simulink model "Hybrid_control_pid_final"  (R2021a)
settings: Solver=ode4  StartTime=0.0  StopTime=2+dt  FixedStep=dt  RelTol=1e-3
libraries: slpidlib x4
settings Model: Creator=Ashut  LastModifiedBy=Ashut

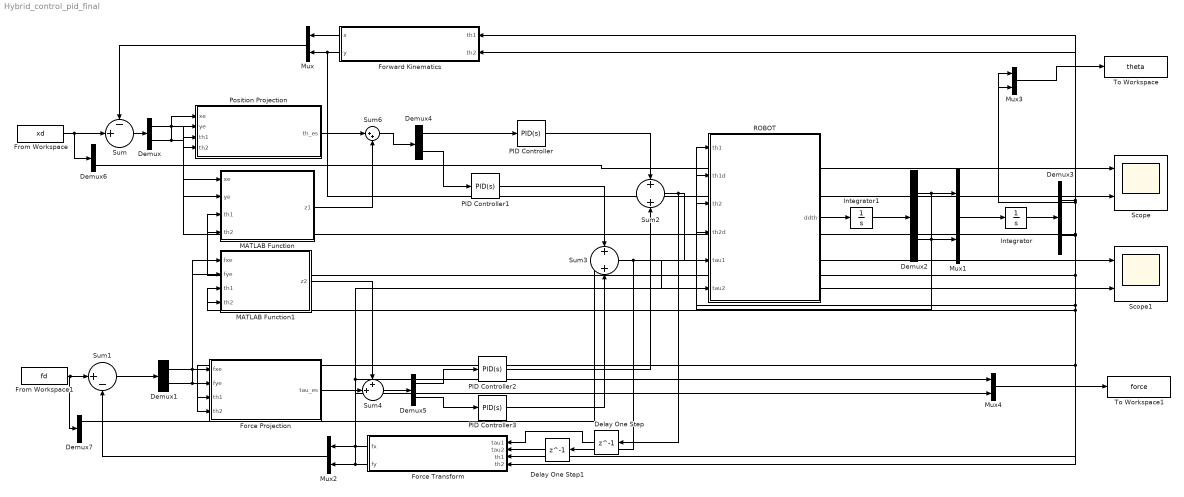
== system Hybrid_control_pid_final ==
  Delay One Step : Delay  DelayLength=1
  Delay One Step1 : Delay  DelayLength=1
  Demux{,1..7} (8 alike) : Demux  Outputs=2
  Force Projection : MATLAB Function  TreatAsAtomicUnit=on
  Force Transform : MATLAB Function  TreatAsAtomicUnit=on
  Forward Kinematics : MATLAB Function  TreatAsAtomicUnit=on
  From Workspace : FromWorkspace  VariableName=xd
  From Workspace1 : FromWorkspace  VariableName=fd
  Integrator : Integrator  InitialCondition=[-pi/3;0]
  Integrator1 : Integrator  InitialCondition=[0;0]
  MATLAB Function : MATLAB Function  TreatAsAtomicUnit=on
  MATLAB Function1 : MATLAB Function  TreatAsAtomicUnit=on
  Mux{,1..4} (5 alike) : Mux  Inputs=2
  PID Controller : slpidlib/PID Controller  Controller=PID  Form=Ideal  TimeDomain=Continuous-time  UseExternalTs=off  SampleTime=-1  IntegratorMethod=Forward Euler  FilterMethod=Forward Euler  ControllerParametersSource=internal  P=1  I=1  D=0  UseFilter=on  N=100  TunerSelectOption=Frequency Response Based  InitialConditionSource=internal  InitialConditionForIntegrator=0  InitialConditionForFilter=0  DifferentiatorICPrevScaledInput=0  ExternalReset=none  TrackingMode=off  Kt=1  LimitOutput=off  SatLimitsSource=internal  UpperSaturationLimit=inf  LowerSaturationLimit=-inf  LinearizeAsGain=on  AntiWindupMode=none  Kb=1  POutMin=[]  POutMax=[]  IOutMin=[]  IOutMax=[]  DOutMin=[]  DOutMax=[]  NOutMin=[]  NOutMax=[]  SumOutMin=[]  SumOutMax=[]  SaturationOutMin=[]  SaturationOutMax=[]  PParamMin=[]  PParamMax=[]  IParamMin=[]  IParamMax=[]  DParamMin=[]  DParamMax=[]  NParamMin=[]  NParamMax=[]  KbParamMin=[]  KbParamMax=[]  KtParamMin=[]  KtParamMax=[]  KbOutMin=[]  KbOutMax=[]  KtOutMin=[]  KtOutMax=[]  IntegratorOutMin=[]  IntegratorOutMax=[]  FilterOutMin=[]  FilterOutMax=[]  SumI1OutMin=[]  SumI1OutMax=[]  SumI2OutMin=[]  SumI2OutMax=[]  SumI3OutMin=[]  SumI3OutMax=[]  SumI4OutMin=[]  SumI4OutMax=[]  SumDOutMin=[]  SumDOutMax=[]  DifferentiatorOutMin=[]  DifferentiatorOutMax=[]  FilterDiffOutCoefMin=[]  FilterDiffOutCoefMax=[]  ReciprocalOutMin=[]  ReciprocalOutMax=[]  SumDenOutMin=[]  SumDenOutMax=[]  SumNumOutMin=[]  SumNumOutMax=[]  DivideOutMin=[]  DivideOutMax=[]  UdiffTsProdOutMin=[]  UdiffTsProdOutMax=[]  NTsProdOutMin=[]  NTsProdOutMax=[]  UintegralTsProdOutMin=[]  UintegralTsProdOutMax=[]  UngainTsProdOutMin=[]  UngainTsProdOutMax=[]  IntegratorContinuousStateAttributes=''  IntegratorStateMustResolveToSignalObject=off  IntegratorRTWStateStorageClass=Auto  FilterContinuousStateAttributes=''  FilterStateMustResolveToSignalObject=off  FilterRTWStateStorageClass=Auto  ParallelPVariant=Passthrough  IdealPVariant=InternalParameters  IVariant=InternalParameters  DVariant=InternalParameters  IntegratorVariant=Continuous  SatVariant=Disabled  AWVariant=Passthrough  PCopyVariant=Disabled  TRVariant=Disabled  FdbkBlocksVariant=Forward  IdealPFdbkVariant=Disabled  SatFdbkVariant=Disabled  DerivativeFilterVariant=ContFilter  NVariant=InternalParameters  NCopyVariant=Disabled  FilterICVariant=InternalICsFilter  IntegratorICVariant=InternalICs  ExternalResetVariant=Disabled  TRSumVariant=Passthrough  SumFdbkVariant=Disabled  SumVariant=Sum_PID  TsampFilterVariant=InternalTs  TsampNgainVariant=Passthrough  TsampIntegralVariant=Passthrough  ExternalSaturationOutDataTypeStr=Inherit: Same as second input
  PID Controller1 : slpidlib/PID Controller  Controller=PID  Form=Ideal  TimeDomain=Continuous-time  UseExternalTs=off  SampleTime=-1  IntegratorMethod=Forward Euler  FilterMethod=Forward Euler  ControllerParametersSource=internal  P=1  I=1  D=0  UseFilter=on  N=100  TunerSelectOption=Transfer Function Based (PID Tuner App)  InitialConditionSource=internal  InitialConditionForIntegrator=0  InitialConditionForFilter=0  DifferentiatorICPrevScaledInput=0  ExternalReset=none  TrackingMode=off  Kt=1  LimitOutput=off  SatLimitsSource=internal  UpperSaturationLimit=inf  LowerSaturationLimit=-inf  LinearizeAsGain=on  AntiWindupMode=none  Kb=1  POutMin=[]  POutMax=[]  IOutMin=[]  IOutMax=[]  DOutMin=[]  DOutMax=[]  NOutMin=[]  NOutMax=[]  SumOutMin=[]  SumOutMax=[]  SaturationOutMin=[]  SaturationOutMax=[]  PParamMin=[]  PParamMax=[]  IParamMin=[]  IParamMax=[]  DParamMin=[]  DParamMax=[]  NParamMin=[]  NParamMax=[]  KbParamMin=[]  KbParamMax=[]  KtParamMin=[]  KtParamMax=[]  KbOutMin=[]  KbOutMax=[]  KtOutMin=[]  KtOutMax=[]  IntegratorOutMin=[]  IntegratorOutMax=[]  FilterOutMin=[]  FilterOutMax=[]  SumI1OutMin=[]  SumI1OutMax=[]  SumI2OutMin=[]  SumI2OutMax=[]  SumI3OutMin=[]  SumI3OutMax=[]  SumI4OutMin=[]  SumI4OutMax=[]  SumDOutMin=[]  SumDOutMax=[]  DifferentiatorOutMin=[]  DifferentiatorOutMax=[]  FilterDiffOutCoefMin=[]  FilterDiffOutCoefMax=[]  ReciprocalOutMin=[]  ReciprocalOutMax=[]  SumDenOutMin=[]  SumDenOutMax=[]  SumNumOutMin=[]  SumNumOutMax=[]  DivideOutMin=[]  DivideOutMax=[]  UdiffTsProdOutMin=[]  UdiffTsProdOutMax=[]  NTsProdOutMin=[]  NTsProdOutMax=[]  UintegralTsProdOutMin=[]  UintegralTsProdOutMax=[]  UngainTsProdOutMin=[]  UngainTsProdOutMax=[]  IntegratorContinuousStateAttributes=''  IntegratorStateMustResolveToSignalObject=off  IntegratorRTWStateStorageClass=Auto  FilterContinuousStateAttributes=''  FilterStateMustResolveToSignalObject=off  FilterRTWStateStorageClass=Auto  ParallelPVariant=Passthrough  IdealPVariant=InternalParameters  IVariant=InternalParameters  DVariant=InternalParameters  IntegratorVariant=Continuous  SatVariant=Disabled  AWVariant=Passthrough  PCopyVariant=Disabled  TRVariant=Disabled  FdbkBlocksVariant=Forward  IdealPFdbkVariant=Disabled  SatFdbkVariant=Disabled  DerivativeFilterVariant=ContFilter  NVariant=InternalParameters  NCopyVariant=Disabled  FilterICVariant=InternalICsFilter  IntegratorICVariant=InternalICs  ExternalResetVariant=Disabled  TRSumVariant=Passthrough  SumFdbkVariant=Disabled  SumVariant=Sum_PID  TsampFilterVariant=InternalTs  TsampNgainVariant=Passthrough  TsampIntegralVariant=Passthrough  ExternalSaturationOutDataTypeStr=Inherit: Same as second input
  PID Controller2 : slpidlib/PID Controller  Controller=PID  Form=Ideal  TimeDomain=Continuous-time  UseExternalTs=off  SampleTime=-1  IntegratorMethod=Forward Euler  FilterMethod=Forward Euler  ControllerParametersSource=internal  P=1  I=1  D=0  UseFilter=on  N=100  TunerSelectOption=Transfer Function Based (PID Tuner App)  InitialConditionSource=internal  InitialConditionForIntegrator=0  InitialConditionForFilter=0  DifferentiatorICPrevScaledInput=0  ExternalReset=none  TrackingMode=off  Kt=1  LimitOutput=off  SatLimitsSource=internal  UpperSaturationLimit=inf  LowerSaturationLimit=-inf  LinearizeAsGain=on  AntiWindupMode=none  Kb=1  POutMin=[]  POutMax=[]  IOutMin=[]  IOutMax=[]  DOutMin=[]  DOutMax=[]  NOutMin=[]  NOutMax=[]  SumOutMin=[]  SumOutMax=[]  SaturationOutMin=[]  SaturationOutMax=[]  PParamMin=[]  PParamMax=[]  IParamMin=[]  IParamMax=[]  DParamMin=[]  DParamMax=[]  NParamMin=[]  NParamMax=[]  KbParamMin=[]  KbParamMax=[]  KtParamMin=[]  KtParamMax=[]  KbOutMin=[]  KbOutMax=[]  KtOutMin=[]  KtOutMax=[]  IntegratorOutMin=[]  IntegratorOutMax=[]  FilterOutMin=[]  FilterOutMax=[]  SumI1OutMin=[]  SumI1OutMax=[]  SumI2OutMin=[]  SumI2OutMax=[]  SumI3OutMin=[]  SumI3OutMax=[]  SumI4OutMin=[]  SumI4OutMax=[]  SumDOutMin=[]  SumDOutMax=[]  DifferentiatorOutMin=[]  DifferentiatorOutMax=[]  FilterDiffOutCoefMin=[]  FilterDiffOutCoefMax=[]  ReciprocalOutMin=[]  ReciprocalOutMax=[]  SumDenOutMin=[]  SumDenOutMax=[]  SumNumOutMin=[]  SumNumOutMax=[]  DivideOutMin=[]  DivideOutMax=[]  UdiffTsProdOutMin=[]  UdiffTsProdOutMax=[]  NTsProdOutMin=[]  NTsProdOutMax=[]  UintegralTsProdOutMin=[]  UintegralTsProdOutMax=[]  UngainTsProdOutMin=[]  UngainTsProdOutMax=[]  IntegratorContinuousStateAttributes=''  IntegratorStateMustResolveToSignalObject=off  IntegratorRTWStateStorageClass=Auto  FilterContinuousStateAttributes=''  FilterStateMustResolveToSignalObject=off  FilterRTWStateStorageClass=Auto  ParallelPVariant=Passthrough  IdealPVariant=InternalParameters  IVariant=InternalParameters  DVariant=InternalParameters  IntegratorVariant=Continuous  SatVariant=Disabled  AWVariant=Passthrough  PCopyVariant=Disabled  TRVariant=Disabled  FdbkBlocksVariant=Forward  IdealPFdbkVariant=Disabled  SatFdbkVariant=Disabled  DerivativeFilterVariant=ContFilter  NVariant=InternalParameters  NCopyVariant=Disabled  FilterICVariant=InternalICsFilter  IntegratorICVariant=InternalICs  ExternalResetVariant=Disabled  TRSumVariant=Passthrough  SumFdbkVariant=Disabled  SumVariant=Sum_PID  TsampFilterVariant=InternalTs  TsampNgainVariant=Passthrough  TsampIntegralVariant=Passthrough  ExternalSaturationOutDataTypeStr=Inherit: Same as second input
  PID Controller3 : slpidlib/PID Controller  Controller=PID  Form=Ideal  TimeDomain=Continuous-time  UseExternalTs=off  SampleTime=-1  IntegratorMethod=Forward Euler  FilterMethod=Forward Euler  ControllerParametersSource=internal  P=1  I=1  D=0  UseFilter=on  N=100  TunerSelectOption=Transfer Function Based (PID Tuner App)  InitialConditionSource=internal  InitialConditionForIntegrator=0  InitialConditionForFilter=0  DifferentiatorICPrevScaledInput=0  ExternalReset=none  TrackingMode=off  Kt=1  LimitOutput=off  SatLimitsSource=internal  UpperSaturationLimit=inf  LowerSaturationLimit=-inf  LinearizeAsGain=on  AntiWindupMode=none  Kb=1  POutMin=[]  POutMax=[]  IOutMin=[]  IOutMax=[]  DOutMin=[]  DOutMax=[]  NOutMin=[]  NOutMax=[]  SumOutMin=[]  SumOutMax=[]  SaturationOutMin=[]  SaturationOutMax=[]  PParamMin=[]  PParamMax=[]  IParamMin=[]  IParamMax=[]  DParamMin=[]  DParamMax=[]  NParamMin=[]  NParamMax=[]  KbParamMin=[]  KbParamMax=[]  KtParamMin=[]  KtParamMax=[]  KbOutMin=[]  KbOutMax=[]  KtOutMin=[]  KtOutMax=[]  IntegratorOutMin=[]  IntegratorOutMax=[]  FilterOutMin=[]  FilterOutMax=[]  SumI1OutMin=[]  SumI1OutMax=[]  SumI2OutMin=[]  SumI2OutMax=[]  SumI3OutMin=[]  SumI3OutMax=[]  SumI4OutMin=[]  SumI4OutMax=[]  SumDOutMin=[]  SumDOutMax=[]  DifferentiatorOutMin=[]  DifferentiatorOutMax=[]  FilterDiffOutCoefMin=[]  FilterDiffOutCoefMax=[]  ReciprocalOutMin=[]  ReciprocalOutMax=[]  SumDenOutMin=[]  SumDenOutMax=[]  SumNumOutMin=[]  SumNumOutMax=[]  DivideOutMin=[]  DivideOutMax=[]  UdiffTsProdOutMin=[]  UdiffTsProdOutMax=[]  NTsProdOutMin=[]  NTsProdOutMax=[]  UintegralTsProdOutMin=[]  UintegralTsProdOutMax=[]  UngainTsProdOutMin=[]  UngainTsProdOutMax=[]  IntegratorContinuousStateAttributes=''  IntegratorStateMustResolveToSignalObject=off  IntegratorRTWStateStorageClass=Auto  FilterContinuousStateAttributes=''  FilterStateMustResolveToSignalObject=off  FilterRTWStateStorageClass=Auto  ParallelPVariant=Passthrough  IdealPVariant=InternalParameters  IVariant=InternalParameters  DVariant=InternalParameters  IntegratorVariant=Continuous  SatVariant=Disabled  AWVariant=Passthrough  PCopyVariant=Disabled  TRVariant=Disabled  FdbkBlocksVariant=Forward  IdealPFdbkVariant=Disabled  SatFdbkVariant=Disabled  DerivativeFilterVariant=ContFilter  NVariant=InternalParameters  NCopyVariant=Disabled  FilterICVariant=InternalICsFilter  IntegratorICVariant=InternalICs  ExternalResetVariant=Disabled  TRSumVariant=Passthrough  SumFdbkVariant=Disabled  SumVariant=Sum_PID  TsampFilterVariant=InternalTs  TsampNgainVariant=Passthrough  TsampIntegralVariant=Passthrough  ExternalSaturationOutDataTypeStr=Inherit: Same as second input
  Position Projection : MATLAB Function  TreatAsAtomicUnit=on
  ROBOT : MATLAB Function  TreatAsAtomicUnit=on
  Scope : Scope  NumInputPorts=2
  Scope1 : Scope  NumInputPorts=2
  Sum : Sum  Inputs=-+|
  Sum1 : Sum  Inputs=|+-
  Sum2 : Sum
  Sum3 : Sum
  Sum4 : Sum  Inputs=++|
  Sum6 : Sum  Inputs=|++
  To Workspace : ToWorkspace  VariableName=theta  SaveFormat=Timeseries  SampleTime=-1
  To Workspace1 : ToWorkspace  VariableName=force  SaveFormat=Timeseries  SampleTime=-1
  wires:
  Mux3/1 -> To Workspace/1
  Mux4/1 -> To Workspace1/1
  Demux/2 -> MATLAB Function/2(ye), Position Projection/2(ye)
  Force Transform/1(fx) -> Mux4/1, Scope1/2, Mux2/1
  ROBOT/1(ddth) -> Integrator1/1
  Demux6/2 -> Scope/1
  Forward Kinematics/2(y) -> Scope/2, Mux/2
  Sum6/1 -> Demux4/1
  Demux7/1 -> Scope1/1
  Delay One Step/1 -> Force Transform/1(tau1)
  Force Transform/2(fy) -> Mux4/2, Mux2/2
  Forward Kinematics/1(x) -> Mux/1
  Mux2/1 -> Sum1/2
  PID Controller2/1 -> Sum2/2
  Delay One Step1/1 -> Force Transform/2(tau2)
  Demux1/1 -> MATLAB Function1/1(fxe), Force Projection/1(fxe)
  MATLAB Function/1(z1) -> Sum6/2
  Mux1/1 -> Integrator/1
  MATLAB Function1/1(z2) -> Sum4/1
  From Workspace/1 -> Demux6/1, Sum/2
  PID Controller1/1 -> Sum3/1
  Demux2/1 -> ROBOT/2(th1d), Mux1/1
  Integrator/1 -> Demux3/1
  From Workspace1/1 -> Demux7/1, Sum1/1
  Demux3/1 -> Force Projection/3(th1), Force Transform/3(th1), MATLAB Function1/3(th1), ROBOT/1(th1), MATLAB Function/3(th1), Position Projection/3(th1), Mux3/1, Forward Kinematics/1(th1)
  Force Projection/1(tau_es) -> Sum4/2
  Demux5/2 -> PID Controller3/1
  Demux5/1 -> PID Controller2/1
  Sum4/1 -> Demux5/1
  Demux1/2 -> MATLAB Function1/2(fye), Force Projection/2(fye)
  Sum2/1 -> Delay One Step/1, ROBOT/5(tau1)
  PID Controller3/1 -> Sum3/2
  Demux2/2 -> ROBOT/4(th2d), Mux1/2
  Sum/1 -> Demux/1
  Mux/1 -> Sum/1
  Position Projection/1(th_es) -> Sum6/1
  Integrator1/1 -> Demux2/1
  Demux3/2 -> Force Projection/4(th2), Force Transform/4(th2), MATLAB Function1/4(th2), ROBOT/3(th2), MATLAB Function/4(th2), Forward Kinematics/2(th2), Mux3/2, Position Projection/4(th2)
  Sum3/1 -> Delay One Step1/1, ROBOT/6(tau2)
  Demux/1 -> MATLAB Function/1(xe), Position Projection/1(xe)
  Sum1/1 -> Demux1/1
  Demux4/2 -> PID Controller1/1
  PID Controller/1 -> Sum2/1
  Demux4/1 -> PID Controller/1

== matlab function Hybrid_control_pid_final/Force Projection ==
  data: fxe input; tau_es output; fye input; th1 input; th2 input
function tau_es = Force_Projection(fxe,fye,th1,th2)


S = [1 0;0 0];

l1=1;l2=1;

J=[-l1*sin(th1) - l2*sin(th1+th2),-l2*sin(th1+th2);l1*cos(th1)+l2*cos(th1+th2),l2*cos(th1+th2)];

f_es = [fxe;fye];

tau_es = (S*J)'*f_es;

== matlab function Hybrid_control_pid_final/Position Projection ==
  data: xe input; th_es output; ye input; th1 input; th2 input
function th_es = Position_Projection(xe,ye,th1,th2)

S = [0 0;0 1];

l1=1;l2=1;

J=[-l1*sin(th1) - l2*sin(th1+th2),-l2*sin(th1+th2);l1*cos(th1)+l2*cos(th1+th2),l2*cos(th1+th2)];

x_es = [xe;ye];

th_es = pinv(S*J)*x_es;

== matlab function Hybrid_control_pid_final/ROBOT ==
  data: th1 input; ddth output; th1d input; th2 input; th2d input; tau1 input; tau2 input
function ddth= ode_solver_script_q1_a(th1,th1d,th2,th2d,tau1,tau2)
x = [th1;th1d;th2;th2d];
%% Input parameters
m2=1; m1=1; l1=1; l2=1; g=9.81;


%% Equation of motion 

%M matrix
M11=((((m1/3) + m2)*l1^2) +((m2/3)*l2^2) + (m2*l1*l2*cos(x(3))));
M12=(m2*(((l2^2)/3) + (0.5*l1*l2*cos(x(3)))));
M21=M12;
M22=((1/3)*m2*l2*l2);

%H matrix
H1 =((-m2*l1*l2*sin(x(3))*x(2)*x(4)) - (0.5*m2*l1*l2*sin(x(3))*x(4)*x(4)));
H2 = (0.5 * m2* l1*l2*sin(x(3))*x(2)*x(2));

%G matrix
G1=( ((((0.5*m1) + m2)*l1*cos(x(1))) + (0.5*m2*l2*cos(x(1)+x(3))))*g);
G2=0.5*m2*l2*cos(x(1)+x(3))*g;



M=[M11 M12;M21 M22];

HG = [H1 + G1; H2 + G2];

T=[tau1; tau2];

%% Equation in terms of acceleration

ddth = (inv(M)) * (T)    ;% Joint  accelaration

== matlab function Hybrid_control_pid_final/Forward Kinematics ==
  data: x output; th1 input; y output; th2 input
function [x,y] = Foward_Kinematics(th1,th2)

l1=1;l2=1;
x=l1*cos(th1) + l2*cos(th1+ th2);
y=l1*sin(th1) + l2*sin(th1+ th2);

== matlab function Hybrid_control_pid_final/Force Transform ==
  data: tau1 input; fx output; tau2 input; fy output; th1 input; th2 input
function [fx,fy] = Force_Transform(tau1,tau2,th1,th2)

l1=1;l2=1;

J=[-l1*sin(th1) - l2*sin(th1+th2),-l2*sin(th1+th2);l1*cos(th1)+l2*cos(th1+th2),l2*cos(th1+th2)];

tau = [tau1;tau2];

f = pinv(J')*tau;

fx = f(1);
fy = f(2);

== matlab function Hybrid_control_pid_final/MATLAB Function ==
  data: xe input; ye input; z1 output; th1 input; th2 input
function z1 = null_projection(xe,ye,th1,th2)

xes = [xe;ye];
l1=1;l2=1;

J=[-l1*sin(th1) - l2*sin(th1+th2),-l2*sin(th1+th2);l1*cos(th1)+l2*cos(th1+th2),l2*cos(th1+th2)];

I = [1 0; 0 1];

z_th = pinv(J)*xes;

z1 = (I - (pinv(J)*J))*z_th;

== matlab function Hybrid_control_pid_final/MATLAB Function1 ==
  data: fxe input; z2 output; fye input; th1 input; th2 input
function z2 = null_projection(fxe,fye,th1,th2)

fes = [fxe;fye];
l1=1;l2=1;

J=[-l1*sin(th1) - l2*sin(th1+th2),-l2*sin(th1+th2);l1*cos(th1)+l2*cos(th1+th2),l2*cos(th1+th2)];

I = [1 0; 0 1];

z_tau = pinv(J)*fes;

z2 = (I - (pinv(J)*J))*z_tau;
